simulink model "ex3_sim1m"  (R2022b)
settings: Solver=ode45  StartTime=0.0  StopTime=1.5  MaxStep=0.0001  RelTol=1e-3
undefined symbols (not defined in the file): DiscIntNeverNeededParam, Kawu, mot, pid, r, Td, Ts, umax
settings Model: Creator=loren  LastModifiedBy=loren
settings DataIOCC: ReturnWorkspaceOutputs=off

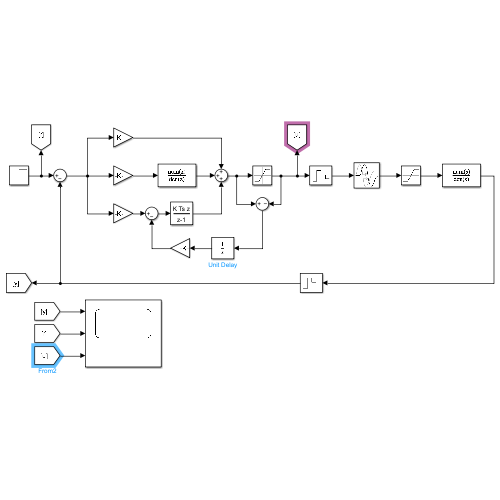
[thumbnail: Simulink's stored preview of the top-level diagram]
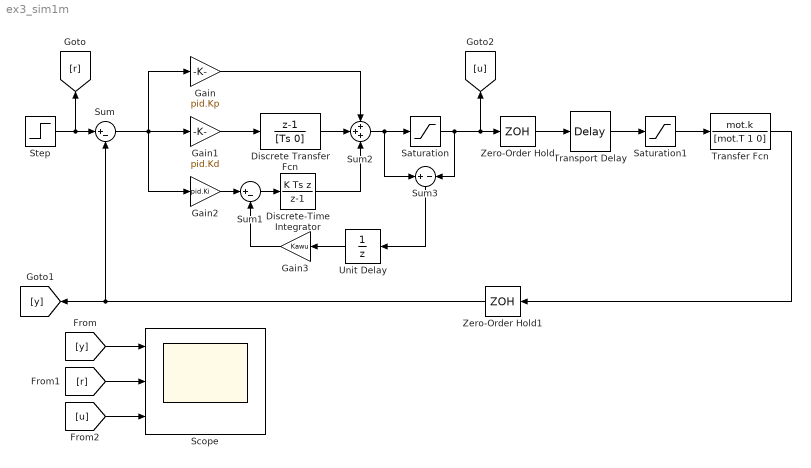
== system ex3_sim1m ==
  Discrete Transfer Fcn : DiscreteTransferFcn  Numerator=[1 -1]  Denominator=[Ts 0]  SampleTime=Ts
  Discrete-Time Integrator : DiscreteIntegrator  IntegratorMethod=Integration: Backward Euler  SampleTime=Ts  ICPrevOutput=DiscIntNeverNeededParam  ICPrevScaledInput=DiscIntNeverNeededParam
  Gain : Gain  Gain=pid.Kp
  Gain1 : Gain  Gain=pid.Kd
  Gain2 : Gain  Gain=pid.Ki
  Gain3 : Gain  Gain=Kawu
  Saturation : Saturate  UpperLimit=umax  LowerLimit=-umax
  Saturation1 : Saturate  UpperLimit=umax  LowerLimit=-umax
  Scope : Scope  NumInputPorts=3
  Step : Step  Time=r.t  After=r.A  SampleTime=0
  Sum : Sum  Inputs=|+-
  Sum1 : Sum  Inputs=|+-
  Sum2 : Sum  Inputs=+++
  Sum3 : Sum  Inputs=+|-
  Transfer Fcn : TransferFcn  Numerator=mot.k  Denominator=[mot.T 1 0]
  Transport Delay : TransportDelay  DelayTime=Td
  Unit Delay : UnitDelay  SampleTime=-1  HasFrameUpgradeWarning=on
  Zero-Order Hold : ZeroOrderHold  SampleTime=Ts
  Zero-Order Hold1 : ZeroOrderHold  SampleTime=Ts
  wires:
  Step/1 -> [r], Sum/1
  Sum/1 -> Gain2/1, Gain1/1, Gain/1
  Gain1/1 -> Discrete Transfer Fcn/1
  Gain2/1 -> Sum1/1
  Sum1/1 -> Discrete-Time Integrator/1
  Gain/1 -> Sum2/1
  Discrete Transfer Fcn/1 -> Sum2/2
  Discrete-Time Integrator/1 -> Sum2/3
  Sum2/1 -> Sum3/1, Saturation/1
  Saturation/1 -> Sum3/2, [u], Zero-Order Hold/1
  Gain3/1 -> Sum1/2
  Unit Delay/1 -> Gain3/1
  Sum3/1 -> Unit Delay/1
  Zero-Order Hold/1 -> Transport Delay/1
  Transport Delay/1 -> Saturation1/1
  Saturation1/1 -> Transfer Fcn/1
  Transfer Fcn/1 -> Zero-Order Hold1/1
  Zero-Order Hold1/1 -> [y], Sum/2
  [y] -> Scope/1
  [r] -> Scope/2
  [u] -> Scope/3
